simulink model "SimulinkFileModel"  (R2023b)
settings: Solver=VariableStepAuto  StartTime=0.0  StopTime=200.0  RelTol=1e-3
values from neighbouring files (symbols this model uses):
  d_r1_t0 = 10^3 * [4.953572247000772; -3.787243278806948; -4.362500902062312]    [MatlabFile.m]
  d_r2_t0 = 10^3 * [5.448929471700850; -4.165967606687643; -4.798750992268544]    [MatlabFile.m]
  epsilon_t0 = 10^(-5)    (= 1e-05)    [MatlabFile.m]
  r1_t0 = 10^6 * [-3.111567646661099; 2.420733547442338; -5.626803092595423]    [MatlabFile.m]
  r2_t0 = 10^6 * [-3.422732421327209; 2.662806902186572; -6.18948308151366]    [MatlabFile.m]
settings Model: Creator=alexa  LastModifiedBy=alexa

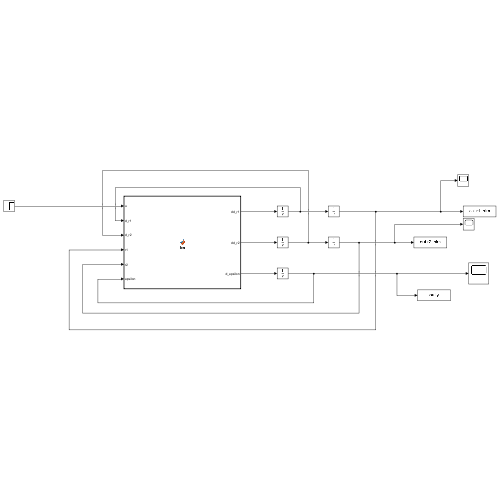
[thumbnail: Simulink's stored preview of the top-level diagram]
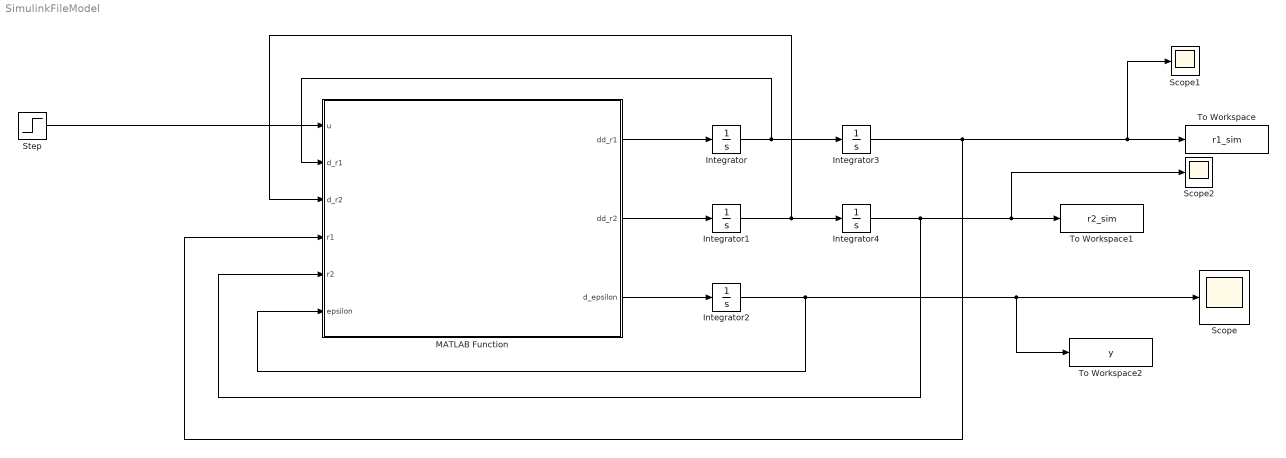
== system SimulinkFileModel ==
  Integrator : Integrator  InitialCondition=d_r1_t0
  Integrator1 : Integrator  InitialCondition=d_r2_t0
  Integrator2 : Integrator  InitialCondition=epsilon_t0
  Integrator3 : Integrator  InitialCondition=r1_t0
  Integrator4 : Integrator  InitialCondition=r2_t0
  MATLAB Function : MATLAB Function  TreatAsAtomicUnit=on
  Scope : Scope
  Scope1 : Scope
  Scope2 : Scope
  Step : Step  Time=2*10^(-3)  SampleTime=0
  To Workspace : ToWorkspace  VariableName=r1_sim  SaveFormat=Timeseries  SampleTime=-1
  To Workspace1 : ToWorkspace  VariableName=r2_sim  SaveFormat=Timeseries  SampleTime=-1
  To Workspace2 : ToWorkspace  VariableName=y  SaveFormat=Timeseries  SampleTime=-1
  wires:
  Step/1 -> MATLAB Function/1(u)
  MATLAB Function/1(dd_r1) -> Integrator/1
  MATLAB Function/2(dd_r2) -> Integrator1/1
  MATLAB Function/3(d_epsilon) -> Integrator2/1
  Integrator/1 -> MATLAB Function/2(d_r1), Integrator3/1
  Integrator1/1 -> MATLAB Function/3(d_r2), Integrator4/1
  Integrator4/1 -> Scope2/1, To Workspace1/1, MATLAB Function/5(r2)
  Integrator2/1 -> MATLAB Function/6(epsilon), To Workspace2/1, Scope/1
  Integrator3/1 -> Scope1/1, To Workspace/1, MATLAB Function/4(r1)

== matlab function SimulinkFileModel/MATLAB Function ==
  data: u input; dd_r1 output; d_r1 input; d_r2 input; r1 input; r2 input; epsilon input; dd_r2 output; d_epsilon output
function [dd_r1,dd_r2,d_epsilon] = fcn(u,d_r1,d_r2,r1,r2,epsilon)

% constants
G = 6.674*10^(-11);
M = 5.972*10^(24); 
R = 6371*10^(3);   
J2 = 1.08262668*10^(-3);
omega = 7.2921*10^(-5);

norm_r1 = norm(r1);
norm_r2 = norm(r2);

g_r1 = -G * M * r1 / norm_r1^3;
g_r1 = g_r1 - (3/2) * (J2 * G * M) * (R^2 / norm_r1^5) * ...
        [r1(1) - 5*r1(1)*r1(3)^2;
         r1(2) - 5*r1(2)*r1(3)^2;
         3*r1(3) - 5*r1(3)^3];
g_r1 = g_r1 + omega^2 * [r1(1); r1(2); 0];
g_r1 = g_r1 + 2 * omega * [d_r1(2); -d_r1(1); 0];

g_r2 = -G * M * r2 / norm_r2^3;
g_r2 = g_r2 - (3/2) * J2 * G * M * R^2 / norm_r2^5 * ...
        [r2(1) - 5*r2(1)*r2(3)^2;
         r2(2) - 5*r2(2)*r2(3)^2;
         3*r2(3) - 5*r2(3)^3];
g_r2 = g_r2 + omega^2 * [r2(1); r2(2); 0];
g_r2 = g_r2 + 2 * omega * [d_r2(2); -d_r2(1); 0];

g_r1 = g_r1 + u;

dd_r1 = g_r1;
dd_r2 = g_r2;

norm_diff = norm(r1 - r2);
d_epsilon = norm_diff / norm_r2;
